simulink model "AircraftPitch"  (R2022a)
settings: Solver=VariableStepAuto  StartTime=0.0  StopTime=10  RelTol=1e-3
settings Model: Creator=teacherforward  LastModifiedBy=teacherforward

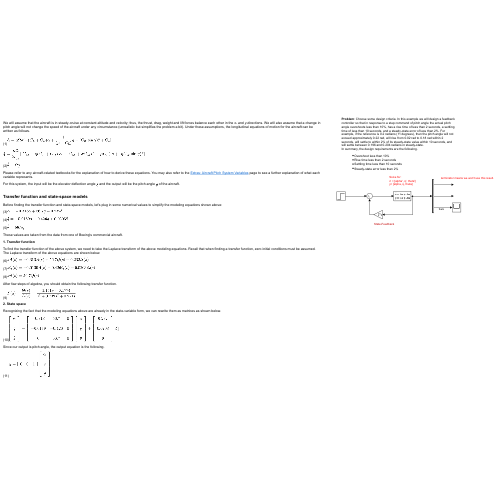
[thumbnail: Simulink's stored preview of the top-level diagram]
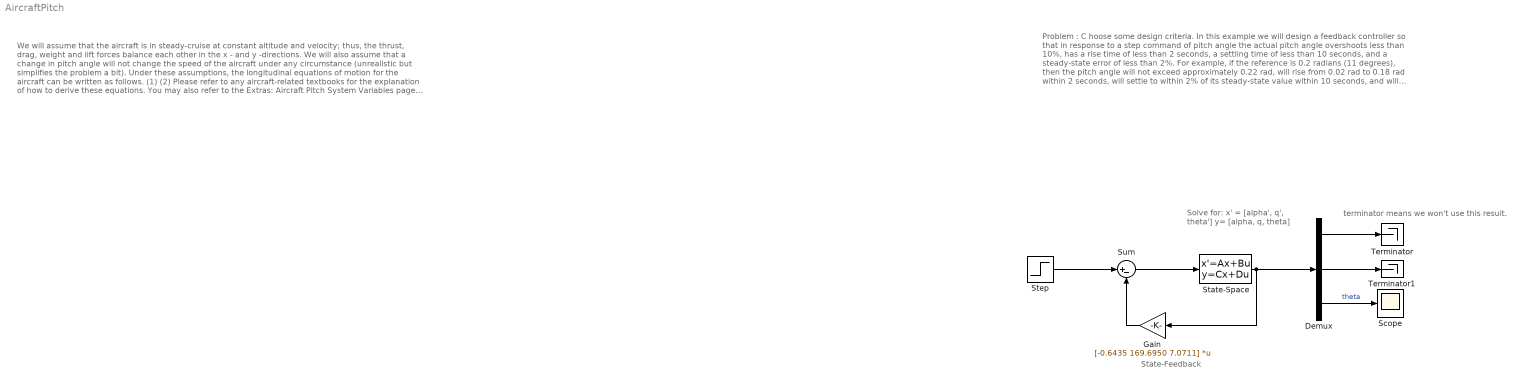
== system AircraftPitch ==
  note: We will assume that the aircraft is in steady-cruise at constant altitude and velocity; thus, the thrust, drag, weight and lift forces balance each other in the x - and y -directions. We will also assume that a change in pitch angle will not change the speed of the aircraft under any circumstance (unrealistic but simplifies the problem a bit). Under these assumptions, the longitudinal equations of motion for the aircraft can be written as follows.
      | (1)
      |
      | (2)
      | Please refer to any aircraft-related textbooks for the explanation of how to derive these equations. You may also refer to the Extras: Aircraft Pitch System Variables page to see a further explanation of what each variable represents.
      | For this system, the input will be the elevator deflection angle and the output will be the pitch angle of the aircraft.
      | Transfer function and state-space models
      | Before finding the transfer function and state-space models, let's plug in some numerical values to simplify the modeling equations shown above:
      | (3)
      | (4)
      | (5)
      | These values are taken from the data from one of Boeing's commercial aircraft.
      | 1. Transfer function
      | To find the transfer function of the above system, we need to take the Laplace transform of the above modeling equations. Recall that when finding a transfer function, zero initial conditions must be assumed. The Laplace transform of the above equations are shown below.
      | (6)
      | (7)
      | (8)
      | After few steps of algebra, you should obtain the following transfer function.
      | (9)
      | 2. State space
      | Recognizing the fact that the modeling equations above are already in the state-variable form, we can rewrite them as matrices as shown below.
      | (10)
      | Since our output is pitch angle, the output equation is the following.
      | (11)
  note: Problem : C hoose some design criteria. In this example we will design a feedback controller so that in response to a step command of pitch angle the actual pitch angle overshoots less than 10%, has a rise time of less than 2 seconds, a settling time of less than 10 seconds, and a steady-state error of less than 2%. For example, if the reference is 0.2 radians (11 degrees), then the pitch angle will not exceed approximately 0.22 rad, will rise from 0.02 rad to 0.18 rad within 2 seconds, will settle to within 2% of its steady-state value within 10 seconds, and will settle between 0.196 and 0.204 radians in steady-state.
      | In summary, the design requirements are the following.
      | Overshoot less than 10%
      | Rise time less than 2 seconds
      | Settling time less than 10 seconds
      | Steady-state error less than 2%
  note: terminator means we won't use this result.
  note: State-Feedback
  note: Solve for:
      | x' = [alpha', q', theta']
      | y= [alpha, q, theta]
  Demux : Demux  Outputs=3
  Gain : Gain  Gain=[-0.6435 169.6950 7.0711]  Multiplication=Matrix(K*u)
  Scope : Scope
  State-Space : StateSpace  A=[-0.313 56.7 0; -0.0139 -0.426 0; 0 56.7 0]  B=[0.232; 0.0203; 0]  C=eye(3)  D=[0;0;0]  InitialCondition=0  ContinuousStateAttributes={'Angle_of_attack', 'Pitch_rate', 'Pitch_angle'}
  Step : Step  Time=0  After=0.2  SampleTime=0
  Sum : Sum  Inputs=|+-
  Terminator : Terminator
  Terminator1 : Terminator
  wires:
  State-Space/1 -> Gain/1, Demux/1
  Demux/2 -> Terminator1/1
  Demux/1 -> Terminator/1
  Demux/3 -> Scope/1  "theta"
  Sum/1 -> State-Space/1
  Gain/1 -> Sum/2
  Step/1 -> Sum/1
